simulink model "REII_312_MyModel"  (R2018b)
settings: Solver=FixedStepDiscrete  StartTime=0.0  StopTime=5  RelTol=1e-3
libraries: dspsnks4 x3, dspvision x2, dspquant2 x1
settings Model: Creator=hermanblackie  LastModifiedBy=adamc
settings SolverCC: AutoInsertRateTranBlk=on
settings DataIOCC: LimitDataPoints=on  SaveOutput=off  SignalLogging=off  SaveTime=off  ReturnWorkspaceOutputs=on
settings OptimizationCC: LifeSpan=inf
settings DebuggingCC: AlgebraicLoopMsg=error  SingleTaskRateTransMsg=error  AllowSymbolicDim=off  SFUnexpectedBacktrackingDiag=warning  SFNoUnconditionalDefaultTransitionDiag=warning  SFExecutionAtInitializationDiag=none
settings SFSimCC: SimUseLocalCustomCode=off
settings RTWCC: RTWUseLocalCustomCode=off
settings CodeAppCC: StateflowObjectComments=on
settings GRTTargetCC: TargetLangStandard=C89/C90 (ANSI)  GeneratePreprocessorConditionals=Disable all
settings ConfigComp: CovMetricSettings=dw  CovHtmlReporting=on  CovSaveCumulativeToWorkspaceVar=on  CovSaveSingleToWorkspaceVar=on  CovExternalEMLEnable=off  CovSFcnEnable=off

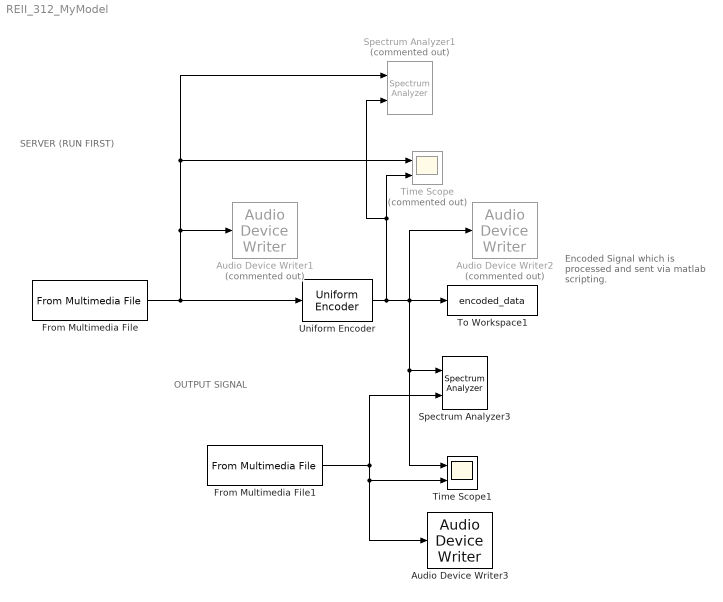
== system REII_312_MyModel ==
  note: SERVER
      | (RUN FIRST)
  note: Encoded Signal which is processed and sent via matlab scripting.
  note: OUTPUT SIGNAL
  Audio Device Writer1 : dspsnks4/Audio Device Writer  Commented=on  Driver=DirectSound  Device=Default  InheritSampleRate=on  SampleRate=44100  BitDepth=16-bit integer  BufferSize=4096  NumBuffers=10  DefaultOutputChannelMapping=on  OutputChannelMapping=1:2  OutputNumUnderrunSamples=off  DriverIdx=1  DeviceWarnFlag=''
  Audio Device Writer2 : dspsnks4/Audio Device Writer  Commented=on  Driver=DirectSound  Device=Default  InheritSampleRate=on  SampleRate=44100  BitDepth=16-bit integer  BufferSize=4096  NumBuffers=10  DefaultOutputChannelMapping=on  OutputChannelMapping=1:2  OutputNumUnderrunSamples=off  DriverIdx=1  DeviceWarnFlag=''
  Audio Device Writer3 : dspsnks4/Audio Device Writer  Driver=DirectSound  Device=Default  InheritSampleRate=on  SampleRate=44100  BitDepth=16-bit integer  BufferSize=4096  NumBuffers=10  DefaultOutputChannelMapping=on  OutputChannelMapping=1:2  OutputNumUnderrunSamples=off  DriverIdx=1  DeviceWarnFlag=''
  From Multimedia File : dspvision/From Multimedia File  inputFilename=C:\Users\adamc\Documents\REII312\prac01\beats.wav  loop=on  numPlays=inf  outputStreams=Audio only  videoDataType=single  audioDataType=double  inheritSampleTime=on  userDefinedSampleTime=1/30  noAudioOutput=off  isIntensityVideo=off  fourcc=RGB  colorVideoFormat=Separate color signals  outputEOF=off  dataOrg=Column-major  audioFrameSize=1024  computeAudioFrameSize=off  outSamplingMode=Sample based
      settings: SourceProductName=DSP System Toolbox  SourceProductBaseCode=DS
  From Multimedia File1 : dspvision/From Multimedia File  inputFilename=C:\Users\adamc\Documents\REII312\prac01\matlab\stereo_output.wav  loop=on  numPlays=inf  outputStreams=Audio only  videoDataType=single  audioDataType=uint8  inheritSampleTime=on  userDefinedSampleTime=1/30  noAudioOutput=off  isIntensityVideo=off  fourcc=RGB  colorVideoFormat=Separate color signals  outputEOF=off  dataOrg=Column-major  audioFrameSize=1024  computeAudioFrameSize=off  outSamplingMode=Sample based
      settings: SourceProductName=DSP System Toolbox  SourceProductBaseCode=DS
  Spectrum Analyzer1 : SpectrumAnalyzer  Commented=on  NumInputPorts=2
  Spectrum Analyzer3 : SpectrumAnalyzer  NumInputPorts=2
  Time Scope : Scope  Commented=on  NumInputPorts=2
  Time Scope1 : Scope  NumInputPorts=2
  To Workspace1 : ToWorkspace  VariableName=encoded_data  SampleTime=-1
      settings: Save2DSignal=2-D array (concatenate along first dimension)
  Uniform Encoder : dspquant2/Uniform Encoder  peak=1  bits=numberOfBits  otype=Unsigned integer
      settings: SourceProductName=DSP System Toolbox
  wires:
  From Multimedia File/1 -> Uniform Encoder/1, Spectrum Analyzer1/1, Time Scope/1, Audio Device Writer1/1
  Uniform Encoder/1 -> Spectrum Analyzer1/2, Time Scope/2, Time Scope1/1, Spectrum Analyzer3/1, Audio Device Writer2/1, To Workspace1/1
  From Multimedia File1/1 -> Audio Device Writer3/1, Time Scope1/2, Spectrum Analyzer3/2
